simulink library "posAugCoef_cl"  (R2022a)
settings: Solver=VariableStepAuto  StartTime=0.0  StopTime=10.0  RelTol=1e-3
undefined symbols (not defined in the file): aRoll, aYaw, azuSweep, bandGap, bRoll, bYaw, DiscIntNeverNeededParam, elevSet, elevStart, env, fftSwitch, FLIGHTCONTROLLER, fltCtrl, fltCtrlPath, FREQ, hiGainTime, initializeBussesFromBlock, intSat, K_filt, lockTime, orientExitTime, orientLaps, pathEstimCtrl, pathLaps, pthCtrl1, rollAmp, rollFreq, rollPhase, rollPow, thetaIGain, thetaPGain, vhcl, yawAmp, yawFreq, yawPhase
libraries: dspsigops x10, slpidlib x5, firstOrderFilter_ul x3, velocityAngle_ul x2, pathFollowingCtrlAoATurb_cl x1, pathFollowingCtrlAoATurbCoef_cl x1, courseFollowLookAhead_cl x1, ctrlAllocMatrix3CompCoef_cl x1, eulAng2RotMat_ul x1, angleBtw2Vecs_ul x1, vrlib x1, alphaBeta_ul x1
(part 1 of 2)
settings Model: Creator=jbfine  LastModifiedBy=jbfine

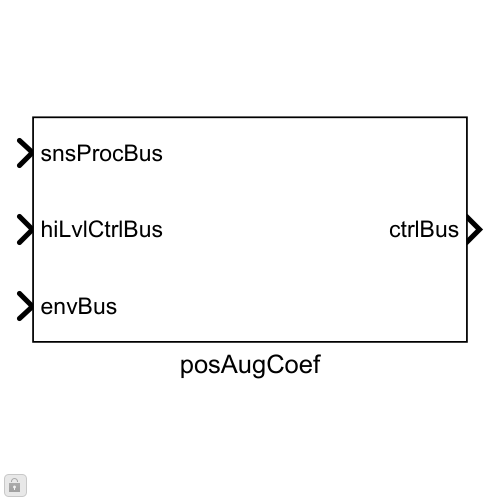
[thumbnail: Simulink's stored preview of the top-level diagram]
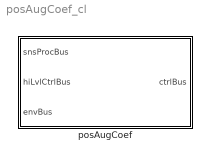
== system posAugCoef_cl ==
  posAugCoef : Subsystem  LoadFcn=initializeBussesFromBlock(gcb)  InitFcn=initializeBussesFromBlock(gcb)  VariantControl="strcmpi(FLIGHTCONTROLLER,\"posAugCoef\")"  mask{initPosForInitSStar=vhcl.initPosVecGnd.Value, fluidDensity=env.water.density.Value, pathCtrl=pthCtrl1, aeroStruct=vhcl.struct('OCT.aeroSurf')}
      mask prompts: initPosForInitSStar "Initial Position"; fluidDensity "Fluid Density"; pathCtrl "Controller"; aeroStruct "Aerodynamic Structure"
      settings: PostSaveFcn=initializeBussesFromBlock(gcb)
      mask DialogControl Container3 Prompt: courseFollow Params
      mask DialogControl Container4 Prompt: setpointToOutput Params

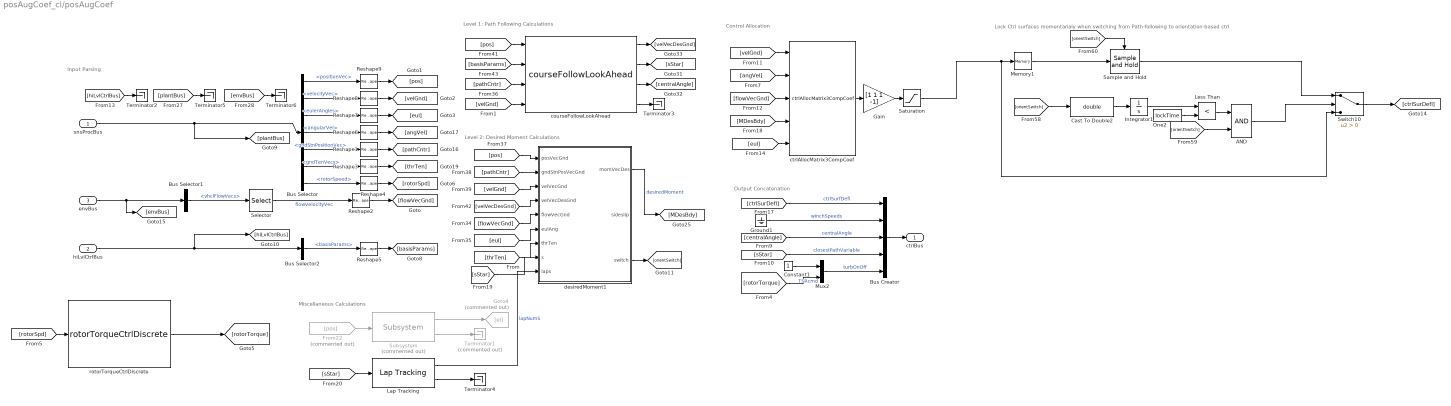
== system posAugCoef_cl/posAugCoef ==
  note: Lock Ctrl surfaces momentarialy when switching from Path-following to orientation-based ctrl
  note: Input Parsing
  note: Control Allocation
  note: Miscellaneous Calculations
  note: Output Concatenation
  note: Level 1: Path Following Calculations
  note: Level 2: Desired Moment Calculations
  snsProcBus : Inport  OutDataTypeStr=Bus: sensorsProcessingBus
  hiLvlCtrlBus : Inport  Port=2
  envBus : Inport  Port=3  OutDataTypeStr=Bus: envBus
  AND : Logic  IconShape=distinctive  AllPortsSameDT=off  OutDataTypeStr=boolean
  Bus Creator : BusCreator  Inputs=5
  Bus Selector : BusSelector  OutputSignals=positionVec,velocityVec,eulerAngles,angularVel,gndStnPositionVec,gndTenVecs,rotorSpeed
  Bus Selector1 : BusSelector  OutputSignals=vhclFlowVecs
  Bus Selector2 : BusSelector  OutputSignals=basisParams
  Cast To Double2 : DataTypeConversion  OutDataTypeStr=double  SaturateOnIntegerOverflow=off  RndMeth=Floor
  Constant1 : Constant
  From22 : From  Commented=on  GotoTag=pos
  Gain : Gain  Gain=[1 1 1 -1]
  Goto4 : Goto  Commented=on  GotoTag=el
  Ground1 : Ground
  Integrator1 : Integrator
  Lap Tracking : pathFollowingCtrlAoATurb_cl/pathFollowingCtrlAoATurb/Lap Tracking  SystemSampleTime=-1  VariantActivationTime=update diagram  Latency=0  AutoFrameSizeCalculation=off
  Less Than : RelationalOperator  Operator=<  OutDataTypeStr=boolean  RndMeth=Simplest  InputSameDT=off
  Memory1 : Memory
  Mux2 : Mux  Inputs=2
  One2 : Constant  Value=lockTime  OutDataTypeStr=Inherit: Inherit via back propagation
  Reshape{1..9} (9 alike) : Reshape  OutputDimensionality=Column vector (2-D)
  Sample and Hold : dspsigops/Sample and Hold  trig=Rising edge  initCond=0  latchinput=off
  Saturation : Saturate  UpperLimit=30  LowerLimit=-30
  Selector : Selector  NumberOfDimensions=2  InputPortWidth=3  IndexOptions=Select all,Index vector (dialog)  Indices=[1 3],5  OutputSizes=1,1
  Subsystem : pathFollowingCtrlAoATurbCoef_cl/pathFollowingCtrlAoATurbCoef/Subsystem  Commented=on  SystemSampleTime=-1  VariantActivationTime=update diagram  Latency=0  AutoFrameSizeCalculation=off
  Switch10 : Switch  Criteria=u2 > Threshold  SaturateOnIntegerOverflow=off  InputSameDT=off
  Terminator1 : Terminator  Commented=on
  Terminator{2..6} (5 alike) : Terminator
  courseFollowLookAhead : courseFollowLookAhead_cl/courseFollowLookAhead  SystemSampleTime=-1  VariantActivationTime=update diagram  Latency=0  AutoFrameSizeCalculation=off
  ctrlAllocMatrix3CompCoef : ctrlAllocMatrix3CompCoef_cl/ctrlAllocMatrix3CompCoef  aeroStruct=vhcl.struct('OCT.aeroSurf')  fluidDensity=fluidDensity  arms=vhcl.struct('OCT.thrAttch')
  desiredMoment1 : Subsystem  AncestorBlock=pathFollowingCtrlAoATurbCoef_cl/pathFollowingCtrlAoATurbCoef/desiredMoment1
  rotorTorqueCtrlDiscrete : rotorTorqueCtrlDiscrete/rotorTorqueCtrlDiscrete  turb_struct=vhcl.struct('OCT.turb')  rho=rho
  ctrlBus : Outport  OutDataTypeStr=Bus: fltCtrlBus  VectorParamsAs1DForOutWhenUnconnected=off
  wires:
  [angVel] -> ctrlAllocMatrix3CompCoef/2
  [pos] -> courseFollowLookAhead/1
  hiLvlCtrlBus/1 -> [hiLvlCtrlBus], Bus Selector2/1
  [pathCntr] -> courseFollowLookAhead/3
  Bus Selector1/1 -> Selector/1  "<vhclFlowVecs>"
  Ground1/1 -> Bus Creator/2  "winchSpeeds"
  Reshape9/1 -> [pos]
  [plantBus] -> Terminator5/1
  Constant1/1 -> Mux2/1
  Lap Tracking/2 -> Terminator4/1
  [sStar] -> Bus Creator/4  "closestPathVariable"
  [flowVecGnd] -> desiredMoment1/5(flowVecGnd)
  Subsystem/2 -> Terminator1/1
  [velGnd] -> courseFollowLookAhead/4
  [sStar] -> desiredMoment1/8(s)
  [velGnd] -> ctrlAllocMatrix3CompCoef/1
  [velVecDesGnd] -> desiredMoment1/4(velVecDesGnd)
  [pos] -> desiredMoment1/1(posVecGnd)
  courseFollowLookAhead/4 -> Terminator3/1
  Reshape4/1 -> [rotorSpd]
  snsProcBus/1 -> [plantBus], Bus Selector/1
  Bus Selector/5 -> Reshape1/1  "<gndStnPositionVec>"
  From22/1 -> Subsystem/1
  [eul] -> desiredMoment1/6(eulAng)
  [basisParams] -> courseFollowLookAhead/2
  Gain/1 -> Saturation/1
  [velGnd] -> desiredMoment1/3(velVecGnd)
  Bus Creator/1 -> ctrlBus/1
  Reshape1/1 -> [pathCntr]
  courseFollowLookAhead/2 -> [sStar]
  envBus/1 -> [envBus], Bus Selector1/1
  Bus Selector2/1 -> Reshape5/1  "<basisParams>"
  Mux2/1 -> Bus Creator/5  "turbOnOff"
  Bus Selector/4 -> Reshape6/1  "<angularVel>"
  [envBus] -> Terminator6/1
  Bus Selector/6 -> Reshape3/1  "<gndTenVecs>"
  courseFollowLookAhead/1 -> [velVecDesGnd]
  Reshape7/1 -> [eul]
  Reshape3/1 -> [thrTen]
  Bus Selector/7 -> Reshape4/1  "<rotorSpeed>"
  desiredMoment1/1(momVecDes) -> [MDesBdy]  "desiredMoment"
  [ctrlSurDefl] -> Bus Creator/1  "ctrlSurfDefl"
  [eul] -> ctrlAllocMatrix3CompCoef/5
  Reshape2/1 -> [flowVecGnd]
  Bus Selector/3 -> Reshape7/1  "<eulerAngles>"
  Reshape5/1 -> [basisParams]
  ctrlAllocMatrix3CompCoef/1 -> Gain/1
  Reshape8/1 -> [velGnd]
  Bus Selector/1 -> Reshape9/1  "<positionVec>"
  Reshape6/1 -> [angVel]
  Subsystem/1 -> Goto4/1
  [centralAngle] -> Bus Creator/3  "centralAngle"
  [sStar] -> Lap Tracking/1
  Selector/1 -> Reshape2/1  "flowVelocityVec"
  Lap Tracking/1 -> desiredMoment1/9(laps)  "lapNumS"
  [rotorSpd] -> rotorTorqueCtrlDiscrete/1
  [MDesBdy] -> ctrlAllocMatrix3CompCoef/4
  courseFollowLookAhead/3 -> [centralAngle]
  [pathCntr] -> desiredMoment1/2(gndStnPosVecGnd)
  [thrTen] -> desiredMoment1/7(thrTen)
  Bus Selector/2 -> Reshape8/1  "<velocityVec>"
  [flowVecGnd] -> ctrlAllocMatrix3CompCoef/3
  [hiLvlCtrlBus] -> Terminator2/1
  rotorTorqueCtrlDiscrete/1 -> [rotorTorque]
  [rotorTorque] -> Mux2/2  "TSRcmd"
  Integrator1/1 -> Less Than/1
  Cast To Double2/1 -> Integrator1/1
  Memory1/1 -> Sample and Hold/1
  Sample and Hold/1 -> Switch10/1
  [orientSwitch] -> AND/2
  [orientSwitch] -> Cast To Double2/1
  One2/1 -> Less Than/2
  [orientSwitch] -> Sample and Hold/Trigger
  Less Than/1 -> AND/1
  AND/1 -> Switch10/2
  Saturation/1 -> Switch10/3, Memory1/1
  Switch10/1 -> [ctrlSurDefl]
  desiredMoment1/3(switch) -> [orientSwitch]

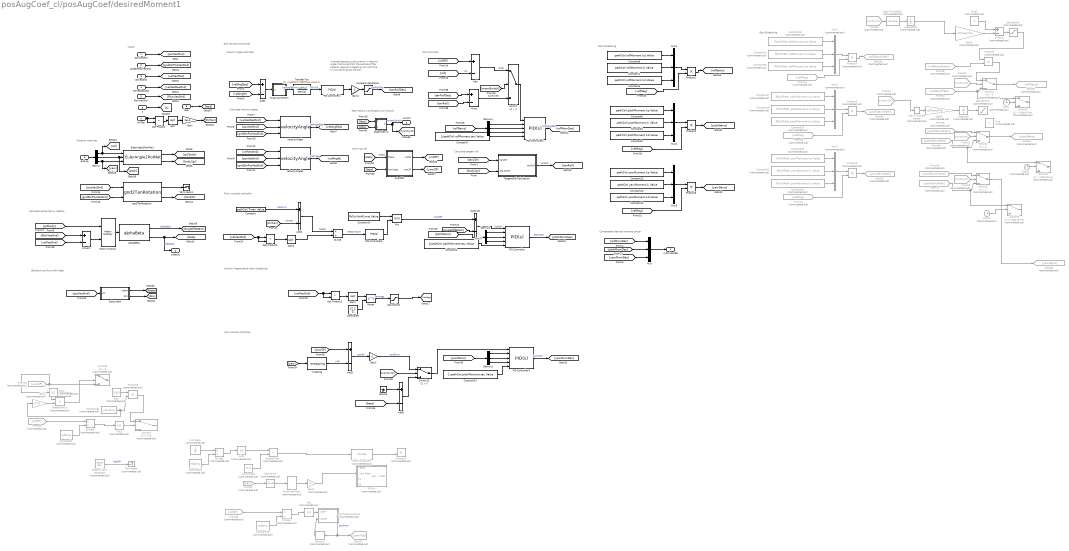
== system posAugCoef_cl/posAugCoef/desiredMoment1 ==
  note: Velocity Magnitude for Gain Scheduling
  note: Roll+Yaw SP
  note: Path-Follow 2 Orientation Ctrl Switch
  note: Elevation and Azimuth Angle
  note: Yaw moment controller
  note: Pitch moment controller
  note: Inverted because a potive error
      | in velocity angle (clockwise from the
      | outside of the sphere) requires a negative
      | roll (With the X-Axis pointing out the tail)
  note: Velocity angle controller
  note: Inputs
  note: Rotation matrices
  note: Calculate velocity angles
  note: Calculate tangent roll
  note: Roll Controller
  note: Concatenate desired moment vector
  note: Calculate aerodynamic sideslip
  note: Roll Moment Controller
  note: Gain Scheduling
  note: Gain Scheduling
  posVecGnd : Inport
  gndStnPosVecGnd : Inport  Port=2
  velVecGnd : Inport  Port=3
  velVecDesGnd : Inport  Port=4
  flowVecGnd : Inport  Port=5
  eulAng : Inport  Port=6
  thrTen : Inport  Port=7
  s : Inport  Port=8
  laps : Inport  Port=9
  Abs{,1..2,4} (4 alike) : Abs  Commented=on  SaturateOnIntegerOverflow=off
  Add{,1..3,5} (5 alike) : Sum  Inputs=+-
  Cast To Double : DataTypeConversion  Commented=on  OutDataTypeStr=double  SaturateOnIntegerOverflow=off  RndMeth=Floor
  Cast To Double1 : DataTypeConversion  Commented=on  OutDataTypeStr=double  SaturateOnIntegerOverflow=off  RndMeth=Floor
  Cast To Double3 : DataTypeConversion  Commented=on  OutDataTypeStr=double  SaturateOnIntegerOverflow=off  RndMeth=Floor
  Clock : Clock  Commented=on
  Clock1 : Clock  Commented=on
  Clock2 : Clock  Commented=on
  Constant : Constant  Value=pathCtrl.Tmax.Value
  Constant1 : Constant  Value=pathCtrl.rollMoment.ki.Value
  Constant10 : Constant  Value=pathCtrl.yawMoment.ki.Value
  Constant11 : Constant  Value=pathCtrl.yawMoment.kd.Value
  Constant12 : Constant  Value=pathCtrl.yawMoment.kp.Value
  Constant13 : Constant  Value=1/pathCtrl.pitchMoment.tau.Value
  Constant14 : Constant  Value=fltCtrl.AoAConst.Value
  Constant16 : Constant  Commented=on  Value=rollAmp
  Constant2 : Constant  Value=pathCtrl.pitchMoment.ki.Value
  Constant20 : Constant  Commented=on  Value=fltCtrlPath.rollMoment.ki.Value
  Constant21 : Constant  Commented=on  Value=fltCtrlPath.yawMoment.ki.Value
  Constant22 : Constant  Commented=on  Value=fltCtrlPath.yawMoment.kd.Value
  Constant23 : Constant  Commented=on  Value=fltCtrlPath.yawMoment.kp.Value
  Constant24 : Constant  Commented=on  Value=fltCtrlPath.pitchMoment.ki.Value
  Constant25 : Constant  Commented=on  Value=fltCtrlPath.pitchMoment.kd.Value
  Constant26 : Constant  Commented=on  Value=fltCtrlPath.rollMoment.kd.Value
  Constant27 : Constant  Commented=on  Value=fltCtrlPath.pitchMoment.kp.Value
  Constant28 : Constant  Commented=on  Value=fltCtrlPath.rollMoment.kp.Value
  Constant29 : Constant  Commented=on  Value=rollAmp
  Constant3 : Constant  Value=pathCtrl.pitchMoment.kd.Value
  Constant30 : Constant  Commented=on  Value=0.5
  Constant31 : Constant  Commented=on  Value=yawAmp
  Constant32 : Constant  Commented=on  Value=rollAmp
  Constant4 : Constant  Value=1/pathCtrl.pitchMoment.tau.Value
  Constant5 : Constant  Value=pathCtrl.rollMoment.kd.Value
  Constant6 : Constant  Value=pathCtrl.pitchMoment.kp.Value
  Constant7 : Constant  Value=1/pathCtrl.rollMoment.tau.Value
  Constant8 : Constant  Value=pathCtrl.rollMoment.kp.Value
  Constant9 : Constant  Value=[2 2 2]
  Demux{,1..3} (4 alike) : Demux  Outputs=3
  Derivative : Derivative  Commented=on
  Divide : Product  Inputs=*/
  Divide1 : Product  Commented=on  Inputs=*/
  Divide2 : Product  Commented=on  Inputs=*/
  Divide3 : Product  Commented=on  Inputs=*/
  Dot Product : DotProduct  OutDataTypeStr=Inherit: Inherit via internal rule
  Dot Product1 : DotProduct  OutDataTypeStr=Inherit: Inherit via internal rule
  Dot Product2 : DotProduct  OutDataTypeStr=Inherit: Inherit via internal rule
  EulerAngle2RotMat1 : eulAng2RotMat_ul/EulerAngle2RotMat  SystemSampleTime=-1  VariantActivationTime=update diagram  Latency=0  AutoFrameSizeCalculation=off
  From39 : From  Commented=on  GotoTag=rollSP
  From40 : From  Commented=on  GotoTag=yawSP
  From42 : From  Commented=on  GotoTag=velMag
  From43 : From  Commented=on  GotoTag=velMag
  From44 : From  Commented=on  GotoTag=velMag
  From45 : From  Commented=on  GotoTag=pitchGainsOrient
  From46 : From  Commented=on  GotoTag=yawGainsOrient
  From47 : From  Commented=on  GotoTag=yawGainsPath
  From48 : From  Commented=on  GotoTag=pitchGainsPath
  From49 : From  Commented=on  GotoTag=rollGainsOrient
  From50 : From  Commented=on  GotoTag=rollGainsPath
  From{51..54,61} (5 alike) : From  Commented=on  GotoTag=orientSwitch
  From55 : From  Commented=on  GotoTag=rollSP
  From57 : From  Commented=on  GotoTag=yaw
  Gain : Gain  Gain=1e-3
  Gain1 : Gain  Gain=-1
  Gain2 : Gain  Gain=-1
  Gain3 : Gain  Commented=on  Gain=rollFreq/4*pi
  Gain4 : Gain  Commented=on  Gain=0.75
  Gain5 : Gain  Commented=on  Gain=-1
  Gain6 : Gain  Commented=on  Gain=-rollFreq/(2*pi)
  Goto32 : Goto  Commented=on  GotoTag=yawMult
  Goto33 : Goto  Commented=on  GotoTag=rollGainsPath
  Goto34 : Goto  Commented=on  GotoTag=pitchGainsPath
  Goto35 : Goto  Commented=on  GotoTag=yawGainsPath
  Goto36 : Goto  Commented=on  GotoTag=rollGains
  Goto38 : Goto  Commented=on  GotoTag=yawGains
  Goto40 : Goto  Commented=on  GotoTag=pitchGains
  GreaterThan : RelationalOperator  Commented=on  Operator=<  OutDataTypeStr=boolean  RndMeth=Simplest  InputSameDT=off
  GreaterThan1 : RelationalOperator  Commented=on  Operator=>  OutDataTypeStr=boolean  RndMeth=Simplest  InputSameDT=off
  Ground : Ground
  Integrator : Integrator  Commented=on
  Integrator2 : Integrator  Commented=on
  MATLAB Function1 : MATLAB Function  Commented=on  TreatAsAtomicUnit=on
  Matrix Multiply : Product  Multiplication=Matrix(*)
  Memory : Memory  Commented=on  InitialCondition=1
  Min : MinMax  Inputs=2
  Minus : Sum  Inputs=+-
  Minus1 : Sum  Inputs=+-
  Minus2 : Sum  Commented=on  Inputs=+-
  Mux{,1..3} (4 alike) : Mux  Inputs=3
  Mux5 : Mux  Commented=on  Inputs=3
  Mux6 : Mux  Commented=on  Inputs=3
  Mux7 : Mux  Commented=on  Inputs=3
  One : Constant  Commented=on  OutDataTypeStr=Inherit: Inherit via back propagation
  One2 : Constant  Commented=on  OutDataTypeStr=Inherit: Inherit via back propagation
  PD ctrl : Subsystem  Commented=on
  PID Controller : slpidlib/PID Controller  Controller=PID  Form=Parallel  TimeDomain=Continuous-time  UseExternalTs=off  SampleTime=-1  IntegratorMethod=Forward Euler  FilterMethod=Forward Euler  ControllerParametersSource=external  P=pathCtrl.pitchMoment.kp.Value  I=pathCtrl.pitchMoment.ki.Value  UseKiTs=off  D=pathCtrl.pitchMoment.kd.Value  N=1/pathCtrl.pitchMoment.tau.Value  UseFilter=on  TunerSelectOption=Transfer Function Based (PID Tuner App)  InitialConditionSource=internal  InitialConditionForIntegrator=0  InitialConditionForFilter=0  DifferentiatorICPrevScaledInput=0  ExternalReset=none  TrackingMode=off  Kt=1  LimitOutput=off  SatLimitsSource=internal  UpperSaturationLimit=inf  LowerSaturationLimit=-100  LinearizeAsGain=on  AntiWindupMode=clamping  Kb=1  POutMin=[]  POutMax=[]  IOutMin=[]  IOutMax=[]  DOutMin=[]  DOutMax=[]  NOutMin=[]  NOutMax=[]  SumOutMin=[]  SumOutMax=[]  SaturationOutMin=[]  SaturationOutMax=[]  PParamMin=[]  PParamMax=[]  IParamMin=[]  IParamMax=[]  DParamMin=[]  DParamMax=[]  NParamMin=[]  NParamMax=[]  KbParamMin=[]  KbParamMax=[]  KtParamMin=[]  KtParamMax=[]  KbOutMin=[]  KbOutMax=[]  KtOutMin=[]  KtOutMax=[]  IntegratorOutMin=[]  IntegratorOutMax=[]  FilterOutMin=[]  FilterOutMax=[]  SumI1OutMin=[]  SumI1OutMax=[]  SumI2OutMin=[]  SumI2OutMax=[]  SumI3OutMin=[]  SumI3OutMax=[]  SumI4OutMin=[]  SumI4OutMax=[]  SumDOutMin=[]  SumDOutMax=[]  DifferentiatorOutMin=[]  DifferentiatorOutMax=[]  FilterDiffOutCoefMin=[]  FilterDiffOutCoefMax=[]  ReciprocalOutMin=[]  ReciprocalOutMax=[]  SumDenOutMin=[]  SumDenOutMax=[]  SumNumOutMin=[]  SumNumOutMax=[]  DivideOutMin=[]  DivideOutMax=[]  UdiffTsProdOutMin=[]  UdiffTsProdOutMax=[]  NTsProdOutMin=[]  NTsProdOutMax=[]  UintegralTsProdOutMin=[]  UintegralTsProdOutMax=[]  UngainTsProdOutMin=[]  UngainTsProdOutMax=[]  IntegratorContinuousStateAttributes=''  IntegratorStateMustResolveToSignalObject=off  IntegratorRTWStateStorageClass=Auto  FilterContinuousStateAttributes=''  FilterStateMustResolveToSignalObject=off  FilterRTWStateStorageClass=Auto  ParallelPVariant=ExternalParameters  IdealPVariant=Disabled  IVariant=ExternalParameters  DVariant=ExternalParameters  IntegratorVariant=Continuous  SatVariant=Disabled  AWVariant=Passthrough  PCopyVariant=Disabled  TRVariant=Disabled  FdbkBlocksVariant=Forward  IdealPFdbkVariant=Disabled  SatFdbkVariant=Disabled  DerivativeFilterVariant=ContFilter  NVariant=ExternalParameters  NCopyVariant=Disabled  FilterICVariant=InternalICsFilter  IntegratorICVariant=InternalICs  ExternalResetVariant=Disabled  TRSumVariant=Passthrough  SumFdbkVariant=Disabled  SumVariant=Sum_PID  TsampFilterVariant=InternalTs  TsampNgainVariant=Passthrough  TsampIntegralVariant=Passthrough  ExternalSaturationOutDataTypeStr=Inherit: Same as second input  aMode=0
  PID Controller1 : slpidlib/PID Controller  Controller=PID  Form=Parallel  TimeDomain=Continuous-time  UseExternalTs=off  SampleTime=-1  IntegratorMethod=Forward Euler  FilterMethod=Forward Euler  ControllerParametersSource=internal  P=pathCtrl.tanRoll.kp.Value  I=pathCtrl.tanRoll.ki.Value  UseKiTs=off  D=pathCtrl.tanRoll.kd.Value  N=1/pathCtrl.tanRoll.tau.Value  UseFilter=on  TunerSelectOption=Transfer Function Based (PID Tuner App)  InitialConditionSource=internal  InitialConditionForIntegrator=0  InitialConditionForFilter=0  DifferentiatorICPrevScaledInput=0  ExternalReset=none  TrackingMode=off  Kt=1  LimitOutput=off  SatLimitsSource=internal  UpperSaturationLimit=inf  LowerSaturationLimit=-100  LinearizeAsGain=on  AntiWindupMode=clamping  Kb=1  POutMin=[]  POutMax=[]  IOutMin=[]  IOutMax=[]  DOutMin=[]  DOutMax=[]  NOutMin=[]  NOutMax=[]  SumOutMin=[]  SumOutMax=[]  SaturationOutMin=[]  SaturationOutMax=[]  PParamMin=[]  PParamMax=[]  IParamMin=[]  IParamMax=[]  DParamMin=[]  DParamMax=[]  NParamMin=[]  NParamMax=[]  KbParamMin=[]  KbParamMax=[]  KtParamMin=[]  KtParamMax=[]  KbOutMin=[]  KbOutMax=[]  KtOutMin=[]  KtOutMax=[]  IntegratorOutMin=[]  IntegratorOutMax=[]  FilterOutMin=[]  FilterOutMax=[]  SumI1OutMin=[]  SumI1OutMax=[]  SumI2OutMin=[]  SumI2OutMax=[]  SumI3OutMin=[]  SumI3OutMax=[]  SumI4OutMin=[]  SumI4OutMax=[]  SumDOutMin=[]  SumDOutMax=[]  DifferentiatorOutMin=[]  DifferentiatorOutMax=[]  FilterDiffOutCoefMin=[]  FilterDiffOutCoefMax=[]  ReciprocalOutMin=[]  ReciprocalOutMax=[]  SumDenOutMin=[]  SumDenOutMax=[]  SumNumOutMin=[]  SumNumOutMax=[]  DivideOutMin=[]  DivideOutMax=[]  UdiffTsProdOutMin=[]  UdiffTsProdOutMax=[]  NTsProdOutMin=[]  NTsProdOutMax=[]  UintegralTsProdOutMin=[]  UintegralTsProdOutMax=[]  UngainTsProdOutMin=[]  UngainTsProdOutMax=[]  IntegratorContinuousStateAttributes=''  IntegratorStateMustResolveToSignalObject=off  IntegratorRTWStateStorageClass=Auto  FilterContinuousStateAttributes=''  FilterStateMustResolveToSignalObject=off  FilterRTWStateStorageClass=Auto  ParallelPVariant=InternalParameters  IdealPVariant=Disabled  IVariant=InternalParameters  DVariant=InternalParameters  IntegratorVariant=Continuous  SatVariant=Disabled  AWVariant=Passthrough  PCopyVariant=Disabled  TRVariant=Disabled  FdbkBlocksVariant=Forward  IdealPFdbkVariant=Disabled  SatFdbkVariant=Disabled  DerivativeFilterVariant=ContFilter  NVariant=InternalParameters  NCopyVariant=Disabled  FilterICVariant=InternalICsFilter  IntegratorICVariant=InternalICs  ExternalResetVariant=Disabled  TRSumVariant=Passthrough  SumFdbkVariant=Disabled  SumVariant=Sum_PID  TsampFilterVariant=InternalTs  TsampNgainVariant=Passthrough  TsampIntegralVariant=Passthrough  ExternalSaturationOutDataTypeStr=Inherit: Same as second input  aMode=0
  PID Controller2 : slpidlib/PID Controller  Controller=PID  Form=Parallel  TimeDomain=Continuous-time  UseExternalTs=off  SampleTime=-1  IntegratorMethod=Forward Euler  FilterMethod=Forward Euler  ControllerParametersSource=external  P=pathCtrl.rollMoment.kp.Value  I=pathCtrl.rollMoment.ki.Value  UseKiTs=off  D=pathCtrl.rollMoment.kd.Value  N=1/pathCtrl.rollMoment.tau.Value  UseFilter=on  TunerSelectOption=Transfer Function Based (PID Tuner App)  InitialConditionSource=internal  InitialConditionForIntegrator=0  InitialConditionForFilter=0  DifferentiatorICPrevScaledInput=0  ExternalReset=none  TrackingMode=off  Kt=1  LimitOutput=off  SatLimitsSource=internal  UpperSaturationLimit=inf  LowerSaturationLimit=-100  LinearizeAsGain=on  AntiWindupMode=clamping  Kb=1  POutMin=[]  POutMax=[]  IOutMin=[]  IOutMax=[]  DOutMin=[]  DOutMax=[]  NOutMin=[]  NOutMax=[]  SumOutMin=[]  SumOutMax=[]  SaturationOutMin=[]  SaturationOutMax=[]  PParamMin=[]  PParamMax=[]  IParamMin=[]  IParamMax=[]  DParamMin=[]  DParamMax=[]  NParamMin=[]  NParamMax=[]  KbParamMin=[]  KbParamMax=[]  KtParamMin=[]  KtParamMax=[]  KbOutMin=[]  KbOutMax=[]  KtOutMin=[]  KtOutMax=[]  IntegratorOutMin=[]  IntegratorOutMax=[]  FilterOutMin=[]  FilterOutMax=[]  SumI1OutMin=[]  SumI1OutMax=[]  SumI2OutMin=[]  SumI2OutMax=[]  SumI3OutMin=[]  SumI3OutMax=[]  SumI4OutMin=[]  SumI4OutMax=[]  SumDOutMin=[]  SumDOutMax=[]  DifferentiatorOutMin=[]  DifferentiatorOutMax=[]  FilterDiffOutCoefMin=[]  FilterDiffOutCoefMax=[]  ReciprocalOutMin=[]  ReciprocalOutMax=[]  SumDenOutMin=[]  SumDenOutMax=[]  SumNumOutMin=[]  SumNumOutMax=[]  DivideOutMin=[]  DivideOutMax=[]  UdiffTsProdOutMin=[]  UdiffTsProdOutMax=[]  NTsProdOutMin=[]  NTsProdOutMax=[]  UintegralTsProdOutMin=[]  UintegralTsProdOutMax=[]  UngainTsProdOutMin=[]  UngainTsProdOutMax=[]  IntegratorContinuousStateAttributes=''  IntegratorStateMustResolveToSignalObject=off  IntegratorRTWStateStorageClass=Auto  FilterContinuousStateAttributes=''  FilterStateMustResolveToSignalObject=off  FilterRTWStateStorageClass=Auto  ParallelPVariant=ExternalParameters  IdealPVariant=Disabled  IVariant=ExternalParameters  DVariant=ExternalParameters  IntegratorVariant=Continuous  SatVariant=Disabled  AWVariant=Passthrough  PCopyVariant=Disabled  TRVariant=Disabled  FdbkBlocksVariant=Forward  IdealPFdbkVariant=Disabled  SatFdbkVariant=Disabled  DerivativeFilterVariant=ContFilter  NVariant=ExternalParameters  NCopyVariant=Disabled  FilterICVariant=InternalICsFilter  IntegratorICVariant=InternalICs  ExternalResetVariant=Disabled  TRSumVariant=Passthrough  SumFdbkVariant=Disabled  SumVariant=Sum_PID  TsampFilterVariant=InternalTs  TsampNgainVariant=Passthrough  TsampIntegralVariant=Passthrough  ExternalSaturationOutDataTypeStr=Inherit: Same as second input  aMode=0
  PID Controller3 : slpidlib/PID Controller  Controller=PID  Form=Parallel  TimeDomain=Continuous-time  UseExternalTs=off  SampleTime=-1  IntegratorMethod=Forward Euler  FilterMethod=Forward Euler  ControllerParametersSource=internal  P=pathCtrl.alphaCtrl.kp.Value  I=pathCtrl.alphaCtrl.ki.Value  UseKiTs=off  D=pathCtrl.alphaCtrl.kd.Value  N=1/pathCtrl.alphaCtrl.tau.Value  UseFilter=on  TunerSelectOption=Transfer Function Based (PID Tuner App)  InitialConditionSource=internal  InitialConditionForIntegrator=0  InitialConditionForFilter=0  DifferentiatorICPrevScaledInput=0  ExternalReset=none  TrackingMode=off  Kt=1  LimitOutput=on  SatLimitsSource=internal  UpperSaturationLimit=pathCtrl.AoAConst.Value+2*pi/180  LowerSaturationLimit=pathCtrl.AoAmin.Value  LinearizeAsGain=on  AntiWindupMode=clamping  Kb=1  POutMin=[]  POutMax=[]  IOutMin=[]  IOutMax=[]  DOutMin=[]  DOutMax=[]  NOutMin=[]  NOutMax=[]  SumOutMin=[]  SumOutMax=[]  SaturationOutMin=[]  SaturationOutMax=[]  PParamMin=[]  PParamMax=[]  IParamMin=[]  IParamMax=[]  DParamMin=[]  DParamMax=[]  NParamMin=[]  NParamMax=[]  KbParamMin=[]  KbParamMax=[]  KtParamMin=[]  KtParamMax=[]  KbOutMin=[]  KbOutMax=[]  KtOutMin=[]  KtOutMax=[]  IntegratorOutMin=[]  IntegratorOutMax=[]  FilterOutMin=[]  FilterOutMax=[]  SumI1OutMin=[]  SumI1OutMax=[]  SumI2OutMin=[]  SumI2OutMax=[]  SumI3OutMin=[]  SumI3OutMax=[]  SumI4OutMin=[]  SumI4OutMax=[]  SumDOutMin=[]  SumDOutMax=[]  DifferentiatorOutMin=[]  DifferentiatorOutMax=[]  FilterDiffOutCoefMin=[]  FilterDiffOutCoefMax=[]  ReciprocalOutMin=[]  ReciprocalOutMax=[]  SumDenOutMin=[]  SumDenOutMax=[]  SumNumOutMin=[]  SumNumOutMax=[]  DivideOutMin=[]  DivideOutMax=[]  UdiffTsProdOutMin=[]  UdiffTsProdOutMax=[]  NTsProdOutMin=[]  NTsProdOutMax=[]  UintegralTsProdOutMin=[]  UintegralTsProdOutMax=[]  UngainTsProdOutMin=[]  UngainTsProdOutMax=[]  IntegratorContinuousStateAttributes=''  IntegratorStateMustResolveToSignalObject=off  IntegratorRTWStateStorageClass=Auto  FilterContinuousStateAttributes=''  FilterStateMustResolveToSignalObject=off  FilterRTWStateStorageClass=Auto  ParallelPVariant=InternalParameters  IdealPVariant=Disabled  IVariant=InternalParameters  DVariant=InternalParameters  IntegratorVariant=Continuous  SatVariant=Enabled  AWVariant=ContClampingParallel  PCopyVariant=Disabled  TRVariant=Disabled  FdbkBlocksVariant=Forward  IdealPFdbkVariant=Disabled  SatFdbkVariant=Disabled  DerivativeFilterVariant=ContFilter  NVariant=InternalParameters  NCopyVariant=Disabled  FilterICVariant=InternalICsFilter  IntegratorICVariant=InternalICs  ExternalResetVariant=Disabled  TRSumVariant=Passthrough  SumFdbkVariant=Disabled  SumVariant=Sum_PID  TsampFilterVariant=InternalTs  TsampNgainVariant=Passthrough  TsampIntegralVariant=Passthrough  ExternalSaturationOutDataTypeStr=Inherit: Same as second input  aMode=0
  PID Controller4 : slpidlib/PID Controller  Controller=PID  Form=Parallel  TimeDomain=Continuous-time  UseExternalTs=off  SampleTime=-1  IntegratorMethod=Forward Euler  FilterMethod=Forward Euler  ControllerParametersSource=external  P=pathCtrl.pitchMoment.kp.Value  I=pathCtrl.pitchMoment.ki.Value  UseKiTs=off  D=pathCtrl.pitchMoment.kd.Value  N=1/pathCtrl.pitchMoment.tau.Value  UseFilter=on  TunerSelectOption=Transfer Function Based (PID Tuner App)  InitialConditionSource=internal  InitialConditionForIntegrator=0  InitialConditionForFilter=0  DifferentiatorICPrevScaledInput=0  ExternalReset=none  TrackingMode=off  Kt=1  LimitOutput=off  SatLimitsSource=internal  UpperSaturationLimit=inf  LowerSaturationLimit=-100  LinearizeAsGain=on  AntiWindupMode=clamping  Kb=1  POutMin=[]  POutMax=[]  IOutMin=[]  IOutMax=[]  DOutMin=[]  DOutMax=[]  NOutMin=[]  NOutMax=[]  SumOutMin=[]  SumOutMax=[]  SaturationOutMin=[]  SaturationOutMax=[]  PParamMin=[]  PParamMax=[]  IParamMin=[]  IParamMax=[]  DParamMin=[]  DParamMax=[]  NParamMin=[]  NParamMax=[]  KbParamMin=[]  KbParamMax=[]  KtParamMin=[]  KtParamMax=[]  KbOutMin=[]  KbOutMax=[]  KtOutMin=[]  KtOutMax=[]  IntegratorOutMin=[]  IntegratorOutMax=[]  FilterOutMin=[]  FilterOutMax=[]  SumI1OutMin=[]  SumI1OutMax=[]  SumI2OutMin=[]  SumI2OutMax=[]  SumI3OutMin=[]  SumI3OutMax=[]  SumI4OutMin=[]  SumI4OutMax=[]  SumDOutMin=[]  SumDOutMax=[]  DifferentiatorOutMin=[]  DifferentiatorOutMax=[]  FilterDiffOutCoefMin=[]  FilterDiffOutCoefMax=[]  ReciprocalOutMin=[]  ReciprocalOutMax=[]  SumDenOutMin=[]  SumDenOutMax=[]  SumNumOutMin=[]  SumNumOutMax=[]  DivideOutMin=[]  DivideOutMax=[]  UdiffTsProdOutMin=[]  UdiffTsProdOutMax=[]  NTsProdOutMin=[]  NTsProdOutMax=[]  UintegralTsProdOutMin=[]  UintegralTsProdOutMax=[]  UngainTsProdOutMin=[]  UngainTsProdOutMax=[]  IntegratorContinuousStateAttributes=''  IntegratorStateMustResolveToSignalObject=off  IntegratorRTWStateStorageClass=Auto  FilterContinuousStateAttributes=''  FilterStateMustResolveToSignalObject=off  FilterRTWStateStorageClass=Auto  ParallelPVariant=ExternalParameters  IdealPVariant=Disabled  IVariant=ExternalParameters  DVariant=ExternalParameters  IntegratorVariant=Continuous  SatVariant=Disabled  AWVariant=Passthrough  PCopyVariant=Disabled  TRVariant=Disabled  FdbkBlocksVariant=Forward  IdealPFdbkVariant=Disabled  SatFdbkVariant=Disabled  DerivativeFilterVariant=ContFilter  NVariant=ExternalParameters  NCopyVariant=Disabled  FilterICVariant=InternalICsFilter  IntegratorICVariant=InternalICs  ExternalResetVariant=Disabled  TRSumVariant=Passthrough  SumFdbkVariant=Disabled  SumVariant=Sum_PID  TsampFilterVariant=InternalTs  TsampNgainVariant=Passthrough  TsampIntegralVariant=Passthrough  ExternalSaturationOutDataTypeStr=Inherit: Same as second input  aMode=0
  Power : Math  Operator=pow
  Product1 : Product
  Product2 : Product
  Product3 : Product
  Product{4..9} (6 alike) : Product  Commented=on
  Saturation1 : Saturate  UpperLimit=100  LowerLimit=0.05
  Saturation2 : Saturate  Commented=on  UpperLimit=1  LowerLimit=3/8
  Saturation3 : Saturate  Commented=on  UpperLimit=1  LowerLimit=1
  Sign : Signum  Commented=on
  Sqrt : Sqrt
  Sqrt1 : Sqrt
  Sqrt2 : Sqrt
  Square Wave Generator : SignalGenerator  Commented=on  WaveForm=square  Amplitude=yawAmp  Frequency=rollFreq  Units=rad/sec
  Subsystem : Subsystem
  Subsystem1 : Subsystem
  Subtract : Sum  Inputs=+-
  Switch : Switch  Criteria=u2 > Threshold  SaturateOnIntegerOverflow=off  InputSameDT=off
  Switch{1..3,9} (4 alike) : Switch  Commented=on  Criteria=u2 > Threshold  SaturateOnIntegerOverflow=off  InputSameDT=off
  Switch11 : Switch  Criteria=u2 > Threshold  SaturateOnIntegerOverflow=off  InputSameDT=off
  Switch4 : Switch  Commented=on  Criteria=u2 > Threshold  Threshold=hiGainTime  SaturateOnIntegerOverflow=off  InputSameDT=off
  Switch5 : Switch  Commented=on  Criteria=u2 > Threshold  Threshold=hiGainTime  SaturateOnIntegerOverflow=off  InputSameDT=off
  Switch6 : Switch  Commented=on  Criteria=u2 > Threshold  Threshold=hiGainTime  SaturateOnIntegerOverflow=off  InputSameDT=off
  Switch7 : Switch  Commented=on  Criteria=u2 > Threshold  Threshold=0.25  SaturateOnIntegerOverflow=off  InputSameDT=off
  TangentRollCalculation : Subsystem
  Terminator : Terminator  Commented=on
  Terminator1 : Terminator
  Transfer Fcn : TransferFcn  Denominator=[pathCtrl.refFiltTau.Value 1]
  Unit Delay : UnitDelay  Commented=on  SampleTime=-1  HasFrameUpgradeWarning=on
  Wrap Correction : Subsystem
  alphaBeta : alphaBeta_ul/alphaBeta  SystemSampleTime=-1  VariantActivationTime=update diagram  Latency=0  AutoFrameSizeCalculation=off
  firstOrderFilter : firstOrderFilter_ul/firstOrderFilter  Commented=on  tau=pathCtrl.pitchMoment.tau.Value  ic=0
  gnd2TanRotation : gnd2TanRotation_ul/gnd2TanRotation  SystemSampleTime=-1  VariantActivationTime=update diagram  Latency=0  AutoFrameSizeCalculation=off
  maxBank Saturation : Saturate  UpperLimit=pathCtrl.maxBank.upperLimit.Value  LowerLimit=pathCtrl.maxBank.lowerLimit.Value
  orientSP : Subsystem  AncestorBlock=posAug_cl/posAug/desiredMoment1/Subsystem
  velocityAngle : velocityAngle_ul/velocityAngle  SystemSampleTime=-1  VariantActivationTime=update diagram  Latency=0  AutoFrameSizeCalculation=off
  velocityAngle1 : velocityAngle_ul/velocityAngle  SystemSampleTime=-1  VariantActivationTime=update diagram  Latency=0  AutoFrameSizeCalculation=off
  wrapping : posAug_cl/posAug/desiredMoment1/wrapping  SystemSampleTime=-1  VariantActivationTime=update diagram  Latency=0  AutoFrameSizeCalculation=off
  momVecDes : Outport  VectorParamsAs1DForOutWhenUnconnected=off
  sideslip : Outport  Port=2
  switch : Outport  Port=3
  wires:
  Saturation1/1 -> [velMag]
  [yaw] -> wrapping/1
  wrapping/1 -> Add3/2  "yaw"
  Add3/1 -> Gain2/1  "yawErr"
  orientSP/1(rollSP) -> [rollSP]
  [theta] -> orientSP/1(theta)  "theta"
  orientSP/2(yawSP) -> [yawSP]
  [posVecGnd] -> Subsystem/1(In1)
  Subsystem/1(theta) -> [theta]
  Constant/1 -> Add2/1  "tensLim"
  Demux3/1 -> PID Controller4/2
  Constant13/1 -> PID Controller4/5
  Demux3/3 -> PID Controller4/4
  Demux3/2 -> PID Controller4/3
  Constant12/1 -> Mux3/1
  Constant11/1 -> Mux3/3
  Constant10/1 -> Mux3/2
  Mux3/1 -> Product3/1
  Product3/1 -> [yawGains]
  [velMag] -> Product3/2
  Sqrt2/1 -> Divide/2
  [velVecGnd] -> Dot Product2/1, Dot Product2/2
  Dot Product2/1 -> Sqrt2/1
  Power/1 -> Saturation1/1  "velmags"
  Constant9/1 -> Power/2
  Sqrt1/1 -> Power/1
  Min/1 -> Subtract/1  "AoASet"
  Demux2/3 -> PID Controller/4
  Demux2/1 -> PID Controller/2
  Demux2/2 -> PID Controller/3
  [velMag] -> Product2/2
  Product2/1 -> [pitchGains]
  Constant3/1 -> Mux2/3
  Constant2/1 -> Mux2/2
  Constant6/1 -> Mux2/1
  Mux2/1 -> Product2/1
  [rollGains] -> Demux1/1
  [velMag] -> Product1/2
  Mux1/1 -> Product1/1
  Constant8/1 -> Mux1/1
  Constant1/1 -> Mux1/2
  Constant5/1 -> Mux1/3
  [velVecGnd] -> Dot Product1/1, Dot Product1/2
  Dot Product1/1 -> Sqrt1/1
  Demux1/2 -> PID Controller2/3
  Constant7/1 -> PID Controller2/5
  Demux1/1 -> PID Controller2/2
  Demux1/3 -> PID Controller2/4
  PID Controller3/1 -> Min/2
  s/1 -> [s]
  Constant4/1 -> PID Controller/5
  Divide/1 -> PID Controller3/1  "TenErrNorm"
  Add2/1 -> Divide/1  "TenErr"
  [thrTen] -> Add2/2  "thrTen"
  Transfer Fcn/1 -> PID Controller1/1  "filtVAE"
  Demux/3 -> EulerAngle2RotMat1/3, [yaw]
  Demux/1 -> EulerAngle2RotMat1/1, [roll]
  Gain/1 -> [thrTen]
  Dot Product/1 -> Sqrt/1
  Sqrt/1 -> Gain/1
  thrTen/1 -> Dot Product/1, Dot Product/2
  Subtract/1 -> PID Controller/1  "AoAerr"
  [angleOfAttack] -> Subtract/2
  PID Controller/1 -> [pitchMomDes]  "elevMom"
  [pitchMomDes] -> Mux/2
  PID Controller1/1 -> Gain1/1
  [yawMomDes] -> Mux/3
  gnd2TanRotation/1 -> Terminator1/1
  gnd2TanRotation/2 -> [tan2Gr]
  [gndStnPosVecGnd] -> gnd2TanRotation/2
  [posVecGnd] -> gnd2TanRotation/1
  [rollSP] -> Add/1
  [roll] -> Add/2  "roll"
  [velVecGnd] -> velocityAngle1/1
  [gndStnPosVecGnd] -> velocityAngle1/3
  [gndStnPosVecGnd] -> velocityAngle/3
  [posVecGnd] -> velocityAngle1/2
  [posVecGnd] -> velocityAngle/2
  [velVecDesGnd] -> velocityAngle/1
  [velAngle] -> Add1/2
  [velAngDes] -> Add1/1
  velocityAngle1/1 -> [velAngle]  "velAngle"
  velocityAngle/1 -> [velAngDes]  "velAngleDes"
  velVecDesGnd/1 -> [velVecDesGnd]
  gndStnPosVecGnd/1 -> [gndStnPosVecGnd]
  alphaBeta/1 -> [angleOfAttack]  "alphaBdy"
  alphaBeta/2 -> sideslip/1, [beta]  "betaBdy"
  Matrix Multiply/1 -> alphaBeta/1
  [gr2body] -> Matrix Multiply/1
  [body2gr] -> TangentRollCalculation/2(bdy2Inert)
  EulerAngle2RotMat1/1 -> [gr2body]
  EulerAngle2RotMat1/2 -> [body2gr]
  Demux/2 -> [pitch], EulerAngle2RotMat1/2
  eulAng/1 -> Demux/1
  [flowVecGnd] -> Minus1/1
  [velVecGnd] -> Minus1/2
  Minus1/1 -> Matrix Multiply/2
  TangentRollCalculation/1(tanRoll) -> [tanRoll]  "tanRoll"
  [tan2Gr] -> TangentRollCalculation/1(tan2Gr)
  flowVecGnd/1 -> [flowVecGnd]
  Add1/1 -> Wrap Correction/1(u)
  maxBank Saturation/1 -> [tanRollDes]  "tanRollDes"
  Gain1/1 -> maxBank Saturation/1
  Add/1 -> Switch/1  "rollEr"
  velVecGnd/1 -> [velVecGnd]
  posVecGnd/1 -> [posVecGnd]
  Wrap Correction/1(y) -> Transfer Fcn/1  "velAngleError"
  [rollMomDes] -> Mux/1
  PID Controller2/1 -> [rollMomDes]  "rollMomDes"
  [pitchGains] -> Demux2/1  "AoASP"
  Subsystem/2(azu) -> [Azu]
  Ground/1 -> Add5/1
  [beta] -> Add5/2
  [tanRollDes] -> Minus/1
  [tanRoll] -> Minus/2
  Minus/1 -> Switch/3  "tanRollErr"
  laps/1 -> [laps]
  Switch/1 -> PID Controller2/1
  [yawGains] -> Demux3/1
  Memory/1 -> MATLAB Function1/2(maxSP)
  From39/1 -> Divide1/1
  MATLAB Function1/1(y) -> Memory/1, Goto32/1  "azuAmp"
  Divide1/1 -> Abs/1
  Constant16/1 -> Divide1/2
  Abs/1 -> MATLAB Function1/1(rollSP)
  Product9/1 -> Switch7/1
  Product1/1 -> [rollGains]
  [Azu] -> Subsystem1/2(azu)
  Subsystem1/1(switch) -> switch/1, [orientSwitch]  "orientSwitch"
  Product4/1 -> Goto33/1
  Constant22/1 -> Mux7/3
  Constant23/1 -> Mux7/1
  Mux6/1 -> Product5/1
  Mux7/1 -> Product6/1
  Constant24/1 -> Mux6/2
  Constant21/1 -> Mux7/2
  From44/1 -> Product6/2
  Constant28/1 -> Mux5/1
  From43/1 -> Product5/2
  Constant25/1 -> Mux6/3
  From42/1 -> Product4/2
  Constant26/1 -> Mux5/3
  Constant27/1 -> Mux6/1
  Product5/1 -> Goto34/1
  Mux5/1 -> Product4/1
  Product6/1 -> Goto35/1
  Constant20/1 -> Mux5/2
  From51/1 -> Switch1/2
  Product7/1 -> Switch1/1
  From50/1 -> Switch4/1, Switch1/3
  From52/1 -> Switch2/2
  From45/1 -> Switch2/1
  From48/1 -> Switch6/1, Switch2/3
  From53/1 -> Switch3/2
  From47/1 -> Switch5/1, Switch3/3
  From46/1 -> Switch3/1
  Clock/1 -> Switch4/2
  Clock1/1 -> Switch5/2
  Clock2/1 -> Switch6/2
  Integrator/1 -> Saturation2/1
  From54/1 -> Cast To Double/1
  Gain3/1 -> Integrator/1
  Cast To Double/1 -> Gain3/1
  Divide2/1 -> Abs1/1
  Constant29/1 -> Divide2/2
  Abs1/1 -> GreaterThan/1
  Constant30/1 -> GreaterThan/2
  GreaterThan/1 -> Cast To Double1/1
  Cast To Double1/1 -> Product8/2
  Unit Delay/1 -> Divide2/1
  Sign/1 -> Product9/1
  Constant31/1 -> Gain4/1, Product9/2
  Abs2/1 -> Switch7/2
  Divide3/1 -> Abs2/1
  Constant32/1 -> Divide3/2
  From55/1 -> Divide3/1
  Square Wave Generator/1 -> Terminator/1  "testSP"
  From40/1 -> Abs4/1, Switch9/3
  GreaterThan1/1 -> Switch9/2
  Abs4/1 -> GreaterThan1/1
  Gain4/1 -> GreaterThan1/2
  [yawSP] -> Add3/1
  From57/1 -> Derivative/1
  Derivative/1 -> firstOrderFilter/1
  Gain5/1 -> PD ctrl/2(- Yaw Rate)
  firstOrderFilter/1 -> Gain5/1
  PID Controller4/1 -> [yawMomDes]  "yawMom"
  Switch3/1 -> Goto38/1
  Switch2/1 -> Goto40/1
  Switch1/1 -> Goto36/1
  Mux/1 -> momVecDes/1
  From61/1 -> Cast To Double3/1
  Cast To Double3/1 -> Integrator2/1
  One2/1 -> Minus2/1
  Integrator2/1 -> Gain6/1
  Minus2/1 -> Saturation3/1
  Gain6/1 -> Minus2/2
  From49/1 -> Product7/2
  Saturation3/1 -> Product7/1
  [laps] -> orientSP/2(numLaps)
  [orientSwitch] -> Switch11/2
  Gain2/1 -> Switch11/1  "yawError"
  Add5/1 -> Switch11/3
  Switch11/1 -> PID Controller4/1
  Constant14/1 -> Min/1
  [laps] -> Subsystem1/1(laps)
  [orientSwitch] -> Switch/2

== system posAugCoef_cl/posAugCoef/desiredMoment1/PD ctrl ==
  - Beta : Inport
  - Yaw Rate : Inport  Port=2
  Kp : Inport  Port=3
  Kd : Inport  Port=4
  Product : Product
  Product1 : Product
  Sum : Sum  Inputs=|++
  yaw Moment Des : Outport
  wires:
  Kd/1 -> Product/2
  - Yaw Rate/1 -> Product/1
  - Beta/1 -> Product1/1
  Kp/1 -> Product1/2
  Product/1 -> Sum/2
  Product1/1 -> Sum/1
  Sum/1 -> yaw Moment Des/1

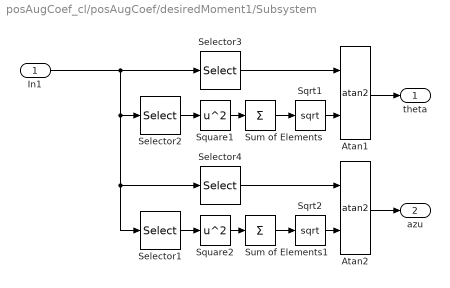
== system posAugCoef_cl/posAugCoef/desiredMoment1/Subsystem ==
  In1 : Inport
  Atan1 : Trigonometry  Operator=atan2
  Atan2 : Trigonometry  Operator=atan2
  Selector1 : Selector  InputPortWidth=3  IndexOptions=Index vector (dialog)  Indices=1  OutputSizes=1
  Selector2 : Selector  InputPortWidth=3  IndexOptions=Index vector (dialog)  Indices=[1 2]  OutputSizes=1
  Selector3 : Selector  InputPortWidth=3  IndexOptions=Index vector (dialog)  Indices=3  OutputSizes=1
  Selector4 : Selector  InputPortWidth=3  IndexOptions=Index vector (dialog)  Indices=2  OutputSizes=1
  Sqrt1 : Sqrt
  Sqrt2 : Sqrt
  Square1 : Math  Operator=square  SignedPower=on
  Square2 : Math  Operator=square  SignedPower=on
  Sum of Elements : Sum  Inputs=+
  Sum of Elements1 : Sum  Inputs=+
  theta : Outport
  azu : Outport  Port=2
  wires:
  Selector3/1 -> Atan1/1
  Sqrt2/1 -> Atan2/2
  Sum of Elements/1 -> Sqrt1/1
  Atan1/1 -> theta/1
  Atan2/1 -> azu/1
  Sqrt1/1 -> Atan1/2
  Square1/1 -> Sum of Elements/1
  Selector2/1 -> Square1/1
  Square2/1 -> Sum of Elements1/1
  Selector1/1 -> Square2/1
  Selector4/1 -> Atan2/1
  In1/1 -> Selector3/1, Selector2/1, Selector4/1, Selector1/1
  Sum of Elements1/1 -> Sqrt2/1

== system posAugCoef_cl/posAugCoef/desiredMoment1/Subsystem1 ==
  laps : Inport
  azu : Inport  Port=2
  AND : Logic  IconShape=distinctive  AllPortsSameDT=off  OutDataTypeStr=boolean
  Abs : Abs  SaturateOnIntegerOverflow=off
  Constant : Constant  Value=0.01
  Constant1 : Constant  Value=pathLaps
  GreaterThan : RelationalOperator  OutDataTypeStr=boolean  RndMeth=Simplest  InputSameDT=off
  Less Than : RelationalOperator  Operator=<  OutDataTypeStr=boolean  RndMeth=Simplest  InputSameDT=off
  Memory : Memory
  OR : Logic  Operator=OR  IconShape=distinctive  AllPortsSameDT=off  OutDataTypeStr=boolean
  switch : Outport
  wires:
  Abs/1 -> Less Than/1
  Constant/1 -> Less Than/2
  Less Than/1 -> AND/2
  laps/1 -> GreaterThan/1
  Constant1/1 -> GreaterThan/2
  GreaterThan/1 -> AND/1
  AND/1 -> OR/2
  OR/1 -> Memory/1, switch/1
  Memory/1 -> OR/1
  azu/1 -> Abs/1

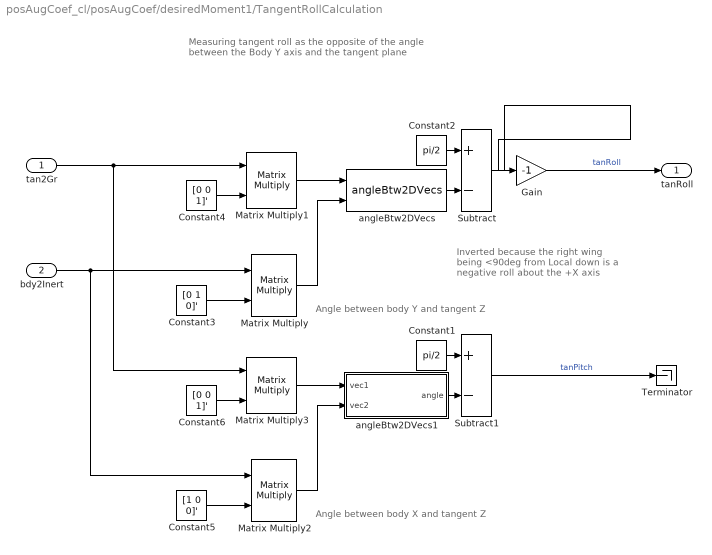
== system posAugCoef_cl/posAugCoef/desiredMoment1/TangentRollCalculation ==
  note: Angle between body X and tangent Z
  note: Inverted because the right wing
      | being <90deg from Local down
      | is a negative roll about the +X axis
  note: Angle between body Y and tangent Z
  note: Measuring tangent roll as the opposite
      | of the angle between the Body Y axis
      | and the tangent plane
  tan2Gr : Inport
  bdy2Inert : Inport  Port=2
  Constant1 : Constant  Value=pi/2
  Constant2 : Constant  Value=pi/2
  Constant3 : Constant  Value=[0 1 0]'
  Constant4 : Constant  Value=[0 0 1]'
  Constant5 : Constant  Value=[1 0 0]'
  Constant6 : Constant  Value=[0 0 1]'
  Gain : Gain  Gain=-1
  Matrix Multiply{,1..3} (4 alike) : Product  Multiplication=Matrix(*)
  Subtract : Sum  Inputs=+-
  Subtract1 : Sum  Inputs=+-
  Terminator : Terminator
  angleBtw2DVecs : angleBtw2Vecs_ul/angleBtw2DVecs  SystemSampleTime=-1  VariantActivationTime=update diagram  Latency=0  AutoFrameSizeCalculation=off
  angleBtw2DVecs1 : Subsystem
  tanRoll : Outport  VectorParamsAs1DForOutWhenUnconnected=off
  wires:
  Constant5/1 -> Matrix Multiply2/2
  angleBtw2DVecs1/1(angle) -> Subtract1/2
  Constant1/1 -> Subtract1/1
  Matrix Multiply3/1 -> angleBtw2DVecs1/1(vec1)
  Constant6/1 -> Matrix Multiply3/2
  Matrix Multiply2/1 -> angleBtw2DVecs1/2(vec2)
  tan2Gr/1 -> Matrix Multiply1/1, Matrix Multiply3/1
  Subtract1/1 -> Terminator/1  "tanPitch"
  bdy2Inert/1 -> Matrix Multiply/1, Matrix Multiply2/1
  Gain/1 -> tanRoll/1  "tanRoll"
  Matrix Multiply/1 -> angleBtw2DVecs/2
  Constant4/1 -> Matrix Multiply1/2
  Matrix Multiply1/1 -> angleBtw2DVecs/1
  Constant2/1 -> Subtract/1
  angleBtw2DVecs/1 -> Subtract/2
  Constant3/1 -> Matrix Multiply/2
  Subtract/1 -> Gain/1

== system posAugCoef_cl/posAugCoef/desiredMoment1/Wrap Correction ==
  note: output = mod(input-pi,2*pi)-pi
      | wraps output to -pi to pi
      |
      | ex) 1.5*pi will become -.5pi
      | 	and -1.5pi will become .5pi
      |
      | to visualize, plot the fuction above
  u : Inport
  Add1 : Sum  Inputs=+-
  Add2 : Sum  Inputs=+-
  Constant1 : Constant  Value=pi
  Constant2 : Constant  Value=2*pi
  Constant3 : Constant  Value=pi
  Mod : Math  Operator=mod  SignedPower=on
  y : Outport  VectorParamsAs1DForOutWhenUnconnected=off
  wires:
  Add2/1 -> y/1
  Constant3/1 -> Add2/2
  Mod/1 -> Add2/1  "always_pos"
  Constant2/1 -> Mod/2
  Add1/1 -> Mod/1
  Constant1/1 -> Add1/2
  u/1 -> Add1/1

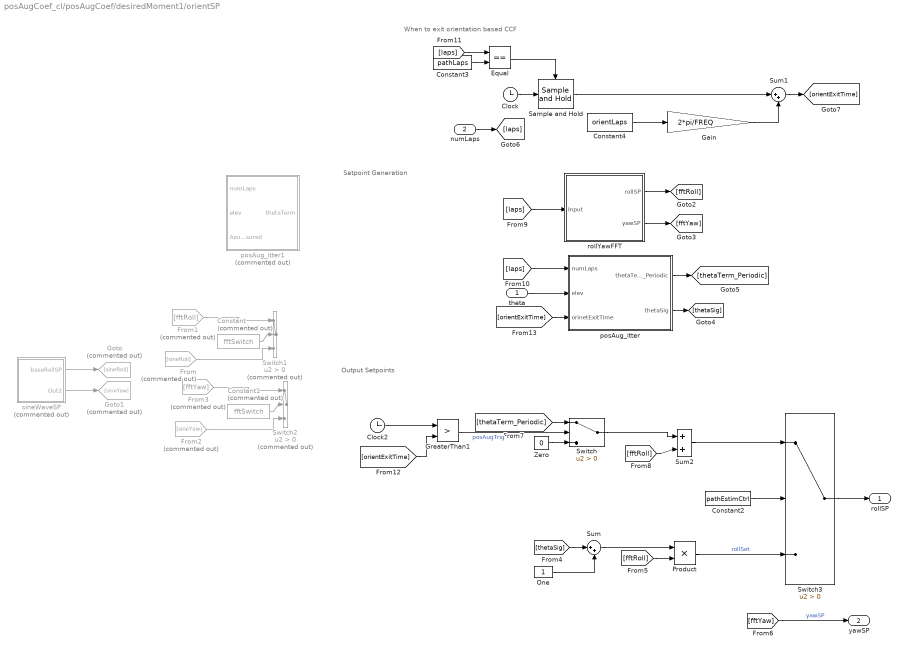
== system posAugCoef_cl/posAugCoef/desiredMoment1/orientSP ==
  note: Setpoint Generation
  note: When to exit orientation based CCF
  note: Output Setpoints
  theta : Inport
  numLaps : Inport  Port=2
  Clock : Clock
  Clock2 : Clock
  Constant : Constant  Commented=on  Value=fftSwitch
  Constant1 : Constant  Commented=on  Value=fftSwitch
  Constant2 : Constant  Value=pathEstimCtrl
  Constant3 : Constant  Value=pathLaps
  Constant4 : Constant  Value=orientLaps
  Equal : RelationalOperator  Operator===  OutDataTypeStr=boolean  RndMeth=Simplest  InputSameDT=off
  From : From  Commented=on  GotoTag=sineRoll
  From1 : From  Commented=on  GotoTag=fftRoll
  From2 : From  Commented=on  GotoTag=sineYaw
  From3 : From  Commented=on  GotoTag=fftYaw
  Gain : Gain  Gain=2*pi/FREQ
  Goto : Goto  Commented=on  GotoTag=sineRoll
  Goto1 : Goto  Commented=on  GotoTag=sineYaw
  GreaterThan1 : RelationalOperator  Operator=>  OutDataTypeStr=boolean  RndMeth=Simplest  InputSameDT=off
  One : Constant  OutDataTypeStr=Inherit: Inherit via back propagation
  Product : Product
  Sample and Hold : dspsigops/Sample and Hold  trig=Rising edge  initCond=10000  latchinput=off
  Sum : Sum  Inputs=|++
  Sum1 : Sum  Inputs=|++
  Sum2 : Sum  Inputs=|++
  Switch : Switch  Criteria=u2 > Threshold  SaturateOnIntegerOverflow=off  InputSameDT=off
  Switch1 : Switch  Commented=on  Criteria=u2 > Threshold  SaturateOnIntegerOverflow=off  InputSameDT=off
  Switch2 : Switch  Commented=on  Criteria=u2 > Threshold  SaturateOnIntegerOverflow=off  InputSameDT=off
  Switch3 : Switch  Criteria=u2 > Threshold  SaturateOnIntegerOverflow=off  InputSameDT=off
  Zero : Constant  Value=0  OutDataTypeStr=Inherit: Inherit via back propagation
  posAug_itter : Subsystem
  posAug_itter1 : Subsystem  Commented=on  AncestorBlock=posAugCoef_cl/posAugCoef/desiredMoment1/orientSP/posAug_itter
  rollYawFFT : Subsystem
  sineWaveSP : Subsystem  Commented=on
  rollSP : Outport
  yawSP : Outport  Port=2
  wires:
  theta/1 -> posAug_itter/2(elev)
  [fftYaw] -> yawSP/1  "yawSP"
  [fftRoll] -> Product/2
  posAug_itter/1(thetaTerm_Periodic) -> [thetaTerm_Periodic]
  Zero/1 -> Switch/3
  [orientExitTime] -> GreaterThan1/2
  GreaterThan1/1 -> Switch/2  "posAugTrig"
  Clock2/1 -> GreaterThan1/1
  sineWaveSP/1(baseRollSP) -> Goto/1
  sineWaveSP/2(Out2) -> Goto1/1
  rollYawFFT/1(rollSP) -> [fftRoll]
  rollYawFFT/2(yawSP) -> [fftYaw]
  Constant/1 -> Switch1/2
  From/1 -> Switch1/3
  From1/1 -> Switch1/1
  From3/1 -> Switch2/1
  From2/1 -> Switch2/3
  Constant1/1 -> Switch2/2
  posAug_itter/2(thetaSig) -> [thetaSig]
  One/1 -> Sum/2
  Sum/1 -> Product/1
  [thetaSig] -> Sum/1
  [thetaTerm_Periodic] -> Switch/1
  [fftRoll] -> Sum2/2
  Switch/1 -> Sum2/1
  Constant2/1 -> Switch3/2
  Sum2/1 -> Switch3/1
  Product/1 -> Switch3/3  "rollSet"
  Switch3/1 -> rollSP/1
  numLaps/1 -> [laps]
  Constant3/1 -> Equal/2
  [laps] -> Equal/1
  Equal/1 -> Sample and Hold/Trigger
  Clock/1 -> Sample and Hold/1
  Sample and Hold/1 -> Sum1/1
  Constant4/1 -> Gain/1
  Gain/1 -> Sum1/2
  [laps] -> rollYawFFT/1(Input)
  [laps] -> posAug_itter/1(numLaps)
  Sum1/1 -> [orientExitTime]
  [orientExitTime] -> posAug_itter/3(orinetExitTime)

== system posAugCoef_cl/posAugCoef/desiredMoment1/TangentRollCalculation/angleBtw2DVecs1 ==
  vec1 : Inport
  vec2 : Inport  Port=2
  Abs : Abs  SaturateOnIntegerOverflow=off
  Atan2 : Trigonometry  Operator=atan2
  Cross Product : vrlib/Utilities/Cross Product
  Dot Product : DotProduct  OutDataTypeStr=Inherit: Inherit via internal rule
  Dot Product1 : DotProduct  OutDataTypeStr=Inherit: Inherit via internal rule
  Sqrt : Sqrt
  angle : Outport  VectorParamsAs1DForOutWhenUnconnected=off
  wires:
  Sqrt/1 -> Atan2/1
  Dot Product1/1 -> Sqrt/1
  Abs/1 -> angle/1
  Dot Product/1 -> Atan2/2
  Cross Product/1 -> Dot Product1/2, Dot Product1/1
  vec2/1 -> Dot Product/2, Cross Product/1
  vec1/1 -> Cross Product/2, Dot Product/1
  Atan2/1 -> Abs/1
